simulink model "Fabregas_et_al"  (R2021b)
settings: Solver=VariableStepAuto  StartTime=0.0  StopTime=60  RelTol=1e-10  AbsTol=1e-14
values from neighbouring files (symbols this model uses):
  q0 = [-0.8;0;pi]    [SIM01.m]    (also in SIM02.m = [j 0 the(k)]'; SIM03.m = [-1;0;-pi/2]; SIM04.m = [1 1 k]'; SIM05.m = [2;1;2])
  s0 = [0;0]    [SIM01.m]    (also in SIM02.m; SIM06.m)
  Thee0 = 0    [SIM01.m]
settings Model: Creator=PC  LastModifiedBy=PC
settings DataIOCC: SaveFormat=Array
settings DebuggingCC: UnderSpecifiedDimensionMsg=warning

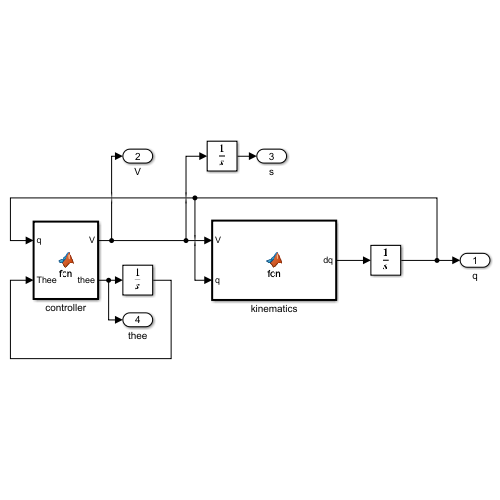
[thumbnail: Simulink's stored preview of the top-level diagram]
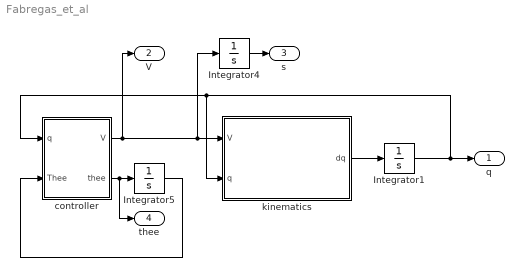
== system Fabregas_et_al ==
  Integrator1 : Integrator  InitialCondition=q0
  Integrator4 : Integrator  InitialCondition=s0
  Integrator5 : Integrator  InitialCondition=Thee0
  controller : MATLAB Function  TreatAsAtomicUnit=on
  kinematics : MATLAB Function  TreatAsAtomicUnit=on
  q : Outport
  V : Outport  Port=2
  s : Outport  Port=3
  thee : Outport  Port=4
  wires:
  controller/1(V) -> V/1, kinematics/1(V), Integrator4/1
  Integrator1/1 -> q/1, kinematics/2(q), controller/1(q)
  Integrator4/1 -> s/1
  controller/2(thee) -> thee/1, Integrator5/1
  Integrator5/1 -> controller/2(Thee)
  kinematics/1(dq) -> Integrator1/1

== matlab function Fabregas_et_al/controller ==
  data: q input size=3*1; V output size=2*1; thee output size=1; Thee input
function [V,thee]= fcn(q,Thee)

the=atan2(sin(q(3)),cos(q(3)));

k1=0.2;kp=0.75;ki=0.00007;
vm=0.05;wm=0.78;

al=atan2(-q(2),-q(1));  
thee=atan2(sin(al-the),cos(al-the));

d=sqrt(q(2)^2+q(1)^2);
v=k1*d*(pi-abs(thee))/pi;
v=min(v,vm);
wd=kp*sin(thee)+ki*Thee;
w=sign(wd)*min(abs(wd),wm);
V=[v;w];

== matlab function Fabregas_et_al/kinematics ==
  data: V input size=2*1; dq output size=3*1; q input size=3*1
function dq = fcn(V,q)
dq=[ cos(q(3))  0
     sin(q(3))  0
      0         1]*V;
